simulink model "boundingbox"  (R2018a)
settings: Solver=VariableStepAuto  StartTime=0.0  StopTime=10.0  RelTol=1e-3
libraries: simulink x128
(part 2 of 4)

== system boundingbox/generate_proximity_sensor_readings/Subsystem/distance_to_bounding_box ==
  note: bounding rectangle
      | C---D
      | |  >  |
      | B---A
  "vertex_a " : Inport
  vertex_b : Inport  Port=2
  vertex_c : Inport  Port=3
  vertex_d : Inport  Port=4
  sensor_pos : Inport  Port=5
  "sensor_ray " : Inport  Port=6
  Inf{,1..3} (4 alike) : Constant  Value=inf
  Min : MinMax  Inputs=4
  Switch{,1..3} (4 alike) : Switch  Criteria=u2 > Threshold
  "calculate_intersection " : Subsystem
  calculate_intersection 1 : Subsystem
  calculate_intersection 2 : Subsystem
  calculate_intersection 3 : Subsystem
  distance : Outport
  wires:
  "vertex_a "/1 -> calculate_intersection 3/2(vertex_2), "calculate_intersection "/1(vertex_1)
  vertex_b/1 -> calculate_intersection 1/1(vertex_1), "calculate_intersection "/2(vertex_2)
  vertex_c/1 -> calculate_intersection 2/1(vertex_1), calculate_intersection 1/2(vertex_2)
  vertex_d/1 -> calculate_intersection 3/1(vertex_1), calculate_intersection 2/2(vertex_2)
  sensor_pos/1 -> calculate_intersection 3/3("origin "), calculate_intersection 2/3("origin "), calculate_intersection 1/3("origin "), "calculate_intersection "/3("origin ")
  "sensor_ray "/1 -> calculate_intersection 3/4(ray), calculate_intersection 2/4(ray), calculate_intersection 1/4(ray), "calculate_intersection "/4(ray)
  "calculate_intersection "/2(intersection (0,1)) -> Switch/2
  Inf/1 -> Switch/3
  Inf1/1 -> Switch1/3
  calculate_intersection 1/2(intersection (0,1)) -> Switch1/2
  calculate_intersection 2/2(intersection (0,1)) -> Switch2/2
  calculate_intersection 3/2(intersection (0,1)) -> Switch3/2
  Inf2/1 -> Switch2/3
  Inf3/1 -> Switch3/3
  calculate_intersection 3/1(distance) -> Switch3/1
  calculate_intersection 2/1(distance) -> Switch2/1
  calculate_intersection 1/1(distance) -> Switch1/1
  "calculate_intersection "/1(distance) -> Switch/1
  Switch/1 -> Min/1
  Switch1/1 -> Min/2
  Switch2/1 -> Min/3
  Switch3/1 -> Min/4
  Min/1 -> distance/1

== system boundingbox/generate_proximity_sensor_readings/Subsystem/distance_to_bounding_box1 ==
  note: bounding rectangle
      | C---D
      | |  >  |
      | B---A
  "vertex_a " : Inport
  vertex_b : Inport  Port=2
  vertex_c : Inport  Port=3
  vertex_d : Inport  Port=4
  sensor_pos : Inport  Port=5
  "sensor_ray " : Inport  Port=6
  Inf{,1..3} (4 alike) : Constant  Value=inf
  Min : MinMax  Inputs=4
  Switch{,1..3} (4 alike) : Switch  Criteria=u2 > Threshold
  "calculate_intersection " : Subsystem
  calculate_intersection 1 : Subsystem
  calculate_intersection 2 : Subsystem
  calculate_intersection 3 : Subsystem
  distance : Outport
  wires:
  Min/1 -> distance/1
  Switch3/1 -> Min/4
  Switch2/1 -> Min/3
  Switch1/1 -> Min/2
  Switch/1 -> Min/1
  "calculate_intersection "/1(distance) -> Switch/1
  calculate_intersection 1/1(distance) -> Switch1/1
  calculate_intersection 2/1(distance) -> Switch2/1
  calculate_intersection 3/1(distance) -> Switch3/1
  Inf3/1 -> Switch3/3
  Inf2/1 -> Switch2/3
  calculate_intersection 3/2(intersection (0,1)) -> Switch3/2
  calculate_intersection 2/2(intersection (0,1)) -> Switch2/2
  calculate_intersection 1/2(intersection (0,1)) -> Switch1/2
  Inf1/1 -> Switch1/3
  Inf/1 -> Switch/3
  "calculate_intersection "/2(intersection (0,1)) -> Switch/2
  "sensor_ray "/1 -> calculate_intersection 3/4(ray), calculate_intersection 2/4(ray), calculate_intersection 1/4(ray), "calculate_intersection "/4(ray)
  sensor_pos/1 -> calculate_intersection 3/3("origin "), calculate_intersection 2/3("origin "), calculate_intersection 1/3("origin "), "calculate_intersection "/3("origin ")
  vertex_d/1 -> calculate_intersection 3/1(vertex_1), calculate_intersection 2/2(vertex_2)
  vertex_c/1 -> calculate_intersection 2/1(vertex_1), calculate_intersection 1/2(vertex_2)
  vertex_b/1 -> calculate_intersection 1/1(vertex_1), "calculate_intersection "/2(vertex_2)
  "vertex_a "/1 -> calculate_intersection 3/2(vertex_2), "calculate_intersection "/1(vertex_1)

== system boundingbox/generate_proximity_sensor_readings/Subsystem/distance_to_bounding_box2 ==
  note: bounding rectangle
      | C---D
      | |  >  |
      | B---A
  "vertex_a " : Inport
  vertex_b : Inport  Port=2
  vertex_c : Inport  Port=3
  vertex_d : Inport  Port=4
  sensor_pos : Inport  Port=5
  "sensor_ray " : Inport  Port=6
  Inf{,1..3} (4 alike) : Constant  Value=inf
  Min : MinMax  Inputs=4
  Switch{,1..3} (4 alike) : Switch  Criteria=u2 > Threshold
  "calculate_intersection " : Subsystem
  calculate_intersection 1 : Subsystem
  calculate_intersection 2 : Subsystem
  calculate_intersection 3 : Subsystem
  distance : Outport
  wires:
  "vertex_a "/1 -> calculate_intersection 3/2(vertex_2), "calculate_intersection "/1(vertex_1)
  vertex_b/1 -> calculate_intersection 1/1(vertex_1), "calculate_intersection "/2(vertex_2)
  vertex_c/1 -> calculate_intersection 2/1(vertex_1), calculate_intersection 1/2(vertex_2)
  vertex_d/1 -> calculate_intersection 3/1(vertex_1), calculate_intersection 2/2(vertex_2)
  sensor_pos/1 -> calculate_intersection 3/3("origin "), calculate_intersection 2/3("origin "), calculate_intersection 1/3("origin "), "calculate_intersection "/3("origin ")
  "sensor_ray "/1 -> calculate_intersection 3/4(ray), calculate_intersection 2/4(ray), calculate_intersection 1/4(ray), "calculate_intersection "/4(ray)
  "calculate_intersection "/2(intersection (0,1)) -> Switch/2
  Inf/1 -> Switch/3
  Inf1/1 -> Switch1/3
  calculate_intersection 1/2(intersection (0,1)) -> Switch1/2
  calculate_intersection 2/2(intersection (0,1)) -> Switch2/2
  calculate_intersection 3/2(intersection (0,1)) -> Switch3/2
  Inf2/1 -> Switch2/3
  Inf3/1 -> Switch3/3
  calculate_intersection 3/1(distance) -> Switch3/1
  calculate_intersection 2/1(distance) -> Switch2/1
  calculate_intersection 1/1(distance) -> Switch1/1
  "calculate_intersection "/1(distance) -> Switch/1
  Switch/1 -> Min/1
  Switch1/1 -> Min/2
  Switch2/1 -> Min/3
  Switch3/1 -> Min/4
  Min/1 -> distance/1

== system boundingbox/generate_proximity_sensor_readings/Subsystem/distance_to_proximity_sensor_data  ==
  distance_cm : Inport
  Constant : Constant  Value=0
  Constant1 : Constant  Value=255
  Gain : Gain  Gain=255/30
  Max : MinMax  Function=max  Inputs=2
  Subtract : Sum  Inputs=+-
  "prox_sensor_input " : Outport
  wires:
  distance_cm/1 -> Gain/1
  Gain/1 -> Subtract/2
  Subtract/1 -> Max/2
  Constant/1 -> Max/1
  Max/1 -> "prox_sensor_input "/1
  Constant1/1 -> Subtract/1

== system boundingbox/generate_proximity_sensor_readings/Subsystem1/distance_to_bounding_box ==
  note: bounding rectangle
      | C---D
      | |  >  |
      | B---A
  "vertex_a " : Inport
  vertex_b : Inport  Port=2
  vertex_c : Inport  Port=3
  vertex_d : Inport  Port=4
  sensor_pos : Inport  Port=5
  "sensor_ray " : Inport  Port=6
  Inf{,1..3} (4 alike) : Constant  Value=inf
  Min : MinMax  Inputs=4
  Switch{,1..3} (4 alike) : Switch  Criteria=u2 > Threshold
  "calculate_intersection " : Subsystem
  calculate_intersection 1 : Subsystem
  calculate_intersection 2 : Subsystem
  calculate_intersection 3 : Subsystem
  distance : Outport
  wires:
  Min/1 -> distance/1
  Switch3/1 -> Min/4
  Switch2/1 -> Min/3
  Switch1/1 -> Min/2
  Switch/1 -> Min/1
  "calculate_intersection "/1(distance) -> Switch/1
  calculate_intersection 1/1(distance) -> Switch1/1
  calculate_intersection 2/1(distance) -> Switch2/1
  calculate_intersection 3/1(distance) -> Switch3/1
  Inf3/1 -> Switch3/3
  Inf2/1 -> Switch2/3
  calculate_intersection 3/2(intersection (0,1)) -> Switch3/2
  calculate_intersection 2/2(intersection (0,1)) -> Switch2/2
  calculate_intersection 1/2(intersection (0,1)) -> Switch1/2
  Inf1/1 -> Switch1/3
  Inf/1 -> Switch/3
  "calculate_intersection "/2(intersection (0,1)) -> Switch/2
  "sensor_ray "/1 -> calculate_intersection 3/4(ray), calculate_intersection 2/4(ray), calculate_intersection 1/4(ray), "calculate_intersection "/4(ray)
  sensor_pos/1 -> calculate_intersection 3/3("origin "), calculate_intersection 2/3("origin "), calculate_intersection 1/3("origin "), "calculate_intersection "/3("origin ")
  vertex_d/1 -> calculate_intersection 3/1(vertex_1), calculate_intersection 2/2(vertex_2)
  vertex_c/1 -> calculate_intersection 2/1(vertex_1), calculate_intersection 1/2(vertex_2)
  vertex_b/1 -> calculate_intersection 1/1(vertex_1), "calculate_intersection "/2(vertex_2)
  "vertex_a "/1 -> calculate_intersection 3/2(vertex_2), "calculate_intersection "/1(vertex_1)

== system boundingbox/generate_proximity_sensor_readings/Subsystem1/distance_to_bounding_box1 ==
  note: bounding rectangle
      | C---D
      | |  >  |
      | B---A
  "vertex_a " : Inport
  vertex_b : Inport  Port=2
  vertex_c : Inport  Port=3
  vertex_d : Inport  Port=4
  sensor_pos : Inport  Port=5
  "sensor_ray " : Inport  Port=6
  Inf{,1..3} (4 alike) : Constant  Value=inf
  Min : MinMax  Inputs=4
  Switch{,1..3} (4 alike) : Switch  Criteria=u2 > Threshold
  "calculate_intersection " : Subsystem
  calculate_intersection 1 : Subsystem
  calculate_intersection 2 : Subsystem
  calculate_intersection 3 : Subsystem
  distance : Outport
  wires:
  "vertex_a "/1 -> calculate_intersection 3/2(vertex_2), "calculate_intersection "/1(vertex_1)
  vertex_b/1 -> calculate_intersection 1/1(vertex_1), "calculate_intersection "/2(vertex_2)
  vertex_c/1 -> calculate_intersection 2/1(vertex_1), calculate_intersection 1/2(vertex_2)
  vertex_d/1 -> calculate_intersection 3/1(vertex_1), calculate_intersection 2/2(vertex_2)
  sensor_pos/1 -> calculate_intersection 3/3("origin "), calculate_intersection 2/3("origin "), calculate_intersection 1/3("origin "), "calculate_intersection "/3("origin ")
  "sensor_ray "/1 -> calculate_intersection 3/4(ray), calculate_intersection 2/4(ray), calculate_intersection 1/4(ray), "calculate_intersection "/4(ray)
  "calculate_intersection "/2(intersection (0,1)) -> Switch/2
  Inf/1 -> Switch/3
  Inf1/1 -> Switch1/3
  calculate_intersection 1/2(intersection (0,1)) -> Switch1/2
  calculate_intersection 2/2(intersection (0,1)) -> Switch2/2
  calculate_intersection 3/2(intersection (0,1)) -> Switch3/2
  Inf2/1 -> Switch2/3
  Inf3/1 -> Switch3/3
  calculate_intersection 3/1(distance) -> Switch3/1
  calculate_intersection 2/1(distance) -> Switch2/1
  calculate_intersection 1/1(distance) -> Switch1/1
  "calculate_intersection "/1(distance) -> Switch/1
  Switch/1 -> Min/1
  Switch1/1 -> Min/2
  Switch2/1 -> Min/3
  Switch3/1 -> Min/4
  Min/1 -> distance/1

== system boundingbox/generate_proximity_sensor_readings/Subsystem1/distance_to_bounding_box2 ==
  note: bounding rectangle
      | C---D
      | |  >  |
      | B---A
  "vertex_a " : Inport
  vertex_b : Inport  Port=2
  vertex_c : Inport  Port=3
  vertex_d : Inport  Port=4
  sensor_pos : Inport  Port=5
  "sensor_ray " : Inport  Port=6
  Inf{,1..3} (4 alike) : Constant  Value=inf
  Min : MinMax  Inputs=4
  Switch{,1..3} (4 alike) : Switch  Criteria=u2 > Threshold
  "calculate_intersection " : Subsystem
  calculate_intersection 1 : Subsystem
  calculate_intersection 2 : Subsystem
  calculate_intersection 3 : Subsystem
  distance : Outport
  wires:
  Min/1 -> distance/1
  Switch3/1 -> Min/4
  Switch2/1 -> Min/3
  Switch1/1 -> Min/2
  Switch/1 -> Min/1
  "calculate_intersection "/1(distance) -> Switch/1
  calculate_intersection 1/1(distance) -> Switch1/1
  calculate_intersection 2/1(distance) -> Switch2/1
  calculate_intersection 3/1(distance) -> Switch3/1
  Inf3/1 -> Switch3/3
  Inf2/1 -> Switch2/3
  calculate_intersection 3/2(intersection (0,1)) -> Switch3/2
  calculate_intersection 2/2(intersection (0,1)) -> Switch2/2
  calculate_intersection 1/2(intersection (0,1)) -> Switch1/2
  Inf1/1 -> Switch1/3
  Inf/1 -> Switch/3
  "calculate_intersection "/2(intersection (0,1)) -> Switch/2
  "sensor_ray "/1 -> calculate_intersection 3/4(ray), calculate_intersection 2/4(ray), calculate_intersection 1/4(ray), "calculate_intersection "/4(ray)
  sensor_pos/1 -> calculate_intersection 3/3("origin "), calculate_intersection 2/3("origin "), calculate_intersection 1/3("origin "), "calculate_intersection "/3("origin ")
  vertex_d/1 -> calculate_intersection 3/1(vertex_1), calculate_intersection 2/2(vertex_2)
  vertex_c/1 -> calculate_intersection 2/1(vertex_1), calculate_intersection 1/2(vertex_2)
  vertex_b/1 -> calculate_intersection 1/1(vertex_1), "calculate_intersection "/2(vertex_2)
  "vertex_a "/1 -> calculate_intersection 3/2(vertex_2), "calculate_intersection "/1(vertex_1)

== system boundingbox/generate_proximity_sensor_readings/Subsystem1/distance_to_proximity_sensor_data  ==
  distance_cm : Inport
  Constant : Constant  Value=0
  Constant1 : Constant  Value=255
  Gain : Gain  Gain=255/30
  Max : MinMax  Function=max  Inputs=2
  Subtract : Sum  Inputs=+-
  "prox_sensor_input " : Outport
  wires:
  Constant1/1 -> Subtract/1
  Max/1 -> "prox_sensor_input "/1
  Constant/1 -> Max/1
  Subtract/1 -> Max/2
  Gain/1 -> Subtract/2
  distance_cm/1 -> Gain/1

== system boundingbox/generate_proximity_sensor_readings/Subsystem2/distance_to_bounding_box ==
  note: bounding rectangle
      | C---D
      | |  >  |
      | B---A
  "vertex_a " : Inport
  vertex_b : Inport  Port=2
  vertex_c : Inport  Port=3
  vertex_d : Inport  Port=4
  sensor_pos : Inport  Port=5
  "sensor_ray " : Inport  Port=6
  Inf{,1..3} (4 alike) : Constant  Value=inf
  Min : MinMax  Inputs=4
  Switch{,1..3} (4 alike) : Switch  Criteria=u2 > Threshold
  "calculate_intersection " : Subsystem
  calculate_intersection 1 : Subsystem
  calculate_intersection 2 : Subsystem
  calculate_intersection 3 : Subsystem
  distance : Outport
  wires:
  "vertex_a "/1 -> calculate_intersection 3/2(vertex_2), "calculate_intersection "/1(vertex_1)
  vertex_b/1 -> calculate_intersection 1/1(vertex_1), "calculate_intersection "/2(vertex_2)
  vertex_c/1 -> calculate_intersection 2/1(vertex_1), calculate_intersection 1/2(vertex_2)
  vertex_d/1 -> calculate_intersection 3/1(vertex_1), calculate_intersection 2/2(vertex_2)
  sensor_pos/1 -> calculate_intersection 3/3("origin "), calculate_intersection 2/3("origin "), calculate_intersection 1/3("origin "), "calculate_intersection "/3("origin ")
  "sensor_ray "/1 -> calculate_intersection 3/4(ray), calculate_intersection 2/4(ray), calculate_intersection 1/4(ray), "calculate_intersection "/4(ray)
  "calculate_intersection "/2(intersection (0,1)) -> Switch/2
  Inf/1 -> Switch/3
  Inf1/1 -> Switch1/3
  calculate_intersection 1/2(intersection (0,1)) -> Switch1/2
  calculate_intersection 2/2(intersection (0,1)) -> Switch2/2
  calculate_intersection 3/2(intersection (0,1)) -> Switch3/2
  Inf2/1 -> Switch2/3
  Inf3/1 -> Switch3/3
  calculate_intersection 3/1(distance) -> Switch3/1
  calculate_intersection 2/1(distance) -> Switch2/1
  calculate_intersection 1/1(distance) -> Switch1/1
  "calculate_intersection "/1(distance) -> Switch/1
  Switch/1 -> Min/1
  Switch1/1 -> Min/2
  Switch2/1 -> Min/3
  Switch3/1 -> Min/4
  Min/1 -> distance/1

== system boundingbox/generate_proximity_sensor_readings/Subsystem2/distance_to_bounding_box1 ==
  note: bounding rectangle
      | C---D
      | |  >  |
      | B---A
  "vertex_a " : Inport
  vertex_b : Inport  Port=2
  vertex_c : Inport  Port=3
  vertex_d : Inport  Port=4
  sensor_pos : Inport  Port=5
  "sensor_ray " : Inport  Port=6
  Inf{,1..3} (4 alike) : Constant  Value=inf
  Min : MinMax  Inputs=4
  Switch{,1..3} (4 alike) : Switch  Criteria=u2 > Threshold
  "calculate_intersection " : Subsystem
  calculate_intersection 1 : Subsystem
  calculate_intersection 2 : Subsystem
  calculate_intersection 3 : Subsystem
  distance : Outport
  wires:
  Min/1 -> distance/1
  Switch3/1 -> Min/4
  Switch2/1 -> Min/3
  Switch1/1 -> Min/2
  Switch/1 -> Min/1
  "calculate_intersection "/1(distance) -> Switch/1
  calculate_intersection 1/1(distance) -> Switch1/1
  calculate_intersection 2/1(distance) -> Switch2/1
  calculate_intersection 3/1(distance) -> Switch3/1
  Inf3/1 -> Switch3/3
  Inf2/1 -> Switch2/3
  calculate_intersection 3/2(intersection (0,1)) -> Switch3/2
  calculate_intersection 2/2(intersection (0,1)) -> Switch2/2
  calculate_intersection 1/2(intersection (0,1)) -> Switch1/2
  Inf1/1 -> Switch1/3
  Inf/1 -> Switch/3
  "calculate_intersection "/2(intersection (0,1)) -> Switch/2
  "sensor_ray "/1 -> calculate_intersection 3/4(ray), calculate_intersection 2/4(ray), calculate_intersection 1/4(ray), "calculate_intersection "/4(ray)
  sensor_pos/1 -> calculate_intersection 3/3("origin "), calculate_intersection 2/3("origin "), calculate_intersection 1/3("origin "), "calculate_intersection "/3("origin ")
  vertex_d/1 -> calculate_intersection 3/1(vertex_1), calculate_intersection 2/2(vertex_2)
  vertex_c/1 -> calculate_intersection 2/1(vertex_1), calculate_intersection 1/2(vertex_2)
  vertex_b/1 -> calculate_intersection 1/1(vertex_1), "calculate_intersection "/2(vertex_2)
  "vertex_a "/1 -> calculate_intersection 3/2(vertex_2), "calculate_intersection "/1(vertex_1)

== system boundingbox/generate_proximity_sensor_readings/Subsystem2/distance_to_bounding_box2 ==
  note: bounding rectangle
      | C---D
      | |  >  |
      | B---A
  "vertex_a " : Inport
  vertex_b : Inport  Port=2
  vertex_c : Inport  Port=3
  vertex_d : Inport  Port=4
  sensor_pos : Inport  Port=5
  "sensor_ray " : Inport  Port=6
  Inf{,1..3} (4 alike) : Constant  Value=inf
  Min : MinMax  Inputs=4
  Switch{,1..3} (4 alike) : Switch  Criteria=u2 > Threshold
  "calculate_intersection " : Subsystem
  calculate_intersection 1 : Subsystem
  calculate_intersection 2 : Subsystem
  calculate_intersection 3 : Subsystem
  distance : Outport
  wires:
  "vertex_a "/1 -> calculate_intersection 3/2(vertex_2), "calculate_intersection "/1(vertex_1)
  vertex_b/1 -> calculate_intersection 1/1(vertex_1), "calculate_intersection "/2(vertex_2)
  vertex_c/1 -> calculate_intersection 2/1(vertex_1), calculate_intersection 1/2(vertex_2)
  vertex_d/1 -> calculate_intersection 3/1(vertex_1), calculate_intersection 2/2(vertex_2)
  sensor_pos/1 -> calculate_intersection 3/3("origin "), calculate_intersection 2/3("origin "), calculate_intersection 1/3("origin "), "calculate_intersection "/3("origin ")
  "sensor_ray "/1 -> calculate_intersection 3/4(ray), calculate_intersection 2/4(ray), calculate_intersection 1/4(ray), "calculate_intersection "/4(ray)
  "calculate_intersection "/2(intersection (0,1)) -> Switch/2
  Inf/1 -> Switch/3
  Inf1/1 -> Switch1/3
  calculate_intersection 1/2(intersection (0,1)) -> Switch1/2
  calculate_intersection 2/2(intersection (0,1)) -> Switch2/2
  calculate_intersection 3/2(intersection (0,1)) -> Switch3/2
  Inf2/1 -> Switch2/3
  Inf3/1 -> Switch3/3
  calculate_intersection 3/1(distance) -> Switch3/1
  calculate_intersection 2/1(distance) -> Switch2/1
  calculate_intersection 1/1(distance) -> Switch1/1
  "calculate_intersection "/1(distance) -> Switch/1
  Switch/1 -> Min/1
  Switch1/1 -> Min/2
  Switch2/1 -> Min/3
  Switch3/1 -> Min/4
  Min/1 -> distance/1

== system boundingbox/generate_proximity_sensor_readings/Subsystem2/distance_to_proximity_sensor_data  ==
  distance_cm : Inport
  Constant : Constant  Value=0
  Constant1 : Constant  Value=255
  Gain : Gain  Gain=255/30
  Max : MinMax  Function=max  Inputs=2
  Subtract : Sum  Inputs=+-
  "prox_sensor_input " : Outport
  wires:
  distance_cm/1 -> Gain/1
  Gain/1 -> Subtract/2
  Subtract/1 -> Max/2
  Constant/1 -> Max/1
  Max/1 -> "prox_sensor_input "/1
  Constant1/1 -> Subtract/1

== system boundingbox/generate_proximity_sensor_readings/bounding_box_CollectorB/vector rotation  ==
  angle : Inport
  x_dir : Inport  Port=2
  y_dir : Inport  Port=3
  Cos : Trigonometry  Operator=cos
  Multiply{,1..3} (4 alike) : Product
  Sin : Trigonometry
  Subtract : Sum  Inputs=+-
  Subtract1 : Sum
  Vector Concatenate1 : Concatenate
  "rotated_vector " : Outport
  wires:
  Multiply2/1 -> Subtract/2
  Subtract/1 -> Vector Concatenate1/1
  Vector Concatenate1/1 -> "rotated_vector "/1
  x_dir/1 -> Multiply/1, Multiply1/1
  angle/1 -> Sin/1, Cos/1
  Sin/1 -> Multiply2/2, Multiply1/2
  Cos/1 -> Multiply/2, Multiply3/2
  Subtract1/1 -> Vector Concatenate1/2
  y_dir/1 -> Multiply2/1, Multiply3/1
  Multiply/1 -> Subtract/1
  Multiply1/1 -> Subtract1/1
  Multiply3/1 -> Subtract1/2

== system boundingbox/generate_proximity_sensor_readings/bounding_box_CollectorB/vector rotation 1 ==
  angle : Inport
  x_dir : Inport  Port=2
  y_dir : Inport  Port=3
  Cos : Trigonometry  Operator=cos
  Multiply{,1..3} (4 alike) : Product
  Sin : Trigonometry
  Subtract : Sum  Inputs=+-
  Subtract1 : Sum
  Vector Concatenate1 : Concatenate
  "rotated_vector " : Outport
  wires:
  Multiply3/1 -> Subtract1/2
  Multiply1/1 -> Subtract1/1
  Multiply/1 -> Subtract/1
  y_dir/1 -> Multiply3/1, Multiply2/1
  Subtract1/1 -> Vector Concatenate1/2
  Cos/1 -> Multiply3/2, Multiply/2
  Sin/1 -> Multiply1/2, Multiply2/2
  angle/1 -> Cos/1, Sin/1
  x_dir/1 -> Multiply1/1, Multiply/1
  Vector Concatenate1/1 -> "rotated_vector "/1
  Subtract/1 -> Vector Concatenate1/1
  Multiply2/1 -> Subtract/2

== system boundingbox/generate_proximity_sensor_readings/bounding_box_ScoutA/vector rotation  ==
  angle : Inport
  x_dir : Inport  Port=2
  y_dir : Inport  Port=3
  Cos : Trigonometry  Operator=cos
  Multiply{,1..3} (4 alike) : Product
  Sin : Trigonometry
  Subtract : Sum  Inputs=+-
  Subtract1 : Sum
  Vector Concatenate1 : Concatenate
  "rotated_vector " : Outport
  wires:
  Multiply2/1 -> Subtract/2
  Subtract/1 -> Vector Concatenate1/1
  Vector Concatenate1/1 -> "rotated_vector "/1
  x_dir/1 -> Multiply/1, Multiply1/1
  angle/1 -> Sin/1, Cos/1
  Sin/1 -> Multiply2/2, Multiply1/2
  Cos/1 -> Multiply/2, Multiply3/2
  Subtract1/1 -> Vector Concatenate1/2
  y_dir/1 -> Multiply2/1, Multiply3/1
  Multiply/1 -> Subtract/1
  Multiply1/1 -> Subtract1/1
  Multiply3/1 -> Subtract1/2

== system boundingbox/generate_proximity_sensor_readings/bounding_box_ScoutA/vector rotation 1 ==
  angle : Inport
  x_dir : Inport  Port=2
  y_dir : Inport  Port=3
  Cos : Trigonometry  Operator=cos
  Multiply{,1..3} (4 alike) : Product
  Sin : Trigonometry
  Subtract : Sum  Inputs=+-
  Subtract1 : Sum
  Vector Concatenate1 : Concatenate
  "rotated_vector " : Outport
  wires:
  Multiply3/1 -> Subtract1/2
  Multiply1/1 -> Subtract1/1
  Multiply/1 -> Subtract/1
  y_dir/1 -> Multiply3/1, Multiply2/1
  Subtract1/1 -> Vector Concatenate1/2
  Cos/1 -> Multiply3/2, Multiply/2
  Sin/1 -> Multiply1/2, Multiply2/2
  angle/1 -> Cos/1, Sin/1
  x_dir/1 -> Multiply1/1, Multiply/1
  Vector Concatenate1/1 -> "rotated_vector "/1
  Subtract/1 -> Vector Concatenate1/1
  Multiply2/1 -> Subtract/2

== system boundingbox/generate_proximity_sensor_readings/bounding_box_ScoutB/vector rotation  ==
  angle : Inport
  x_dir : Inport  Port=2
  y_dir : Inport  Port=3
  Cos : Trigonometry  Operator=cos
  Multiply{,1..3} (4 alike) : Product
  Sin : Trigonometry
  Subtract : Sum  Inputs=+-
  Subtract1 : Sum
  Vector Concatenate1 : Concatenate
  "rotated_vector " : Outport
  wires:
  Multiply3/1 -> Subtract1/2
  Multiply1/1 -> Subtract1/1
  Multiply/1 -> Subtract/1
  y_dir/1 -> Multiply3/1, Multiply2/1
  Subtract1/1 -> Vector Concatenate1/2
  Cos/1 -> Multiply3/2, Multiply/2
  Sin/1 -> Multiply1/2, Multiply2/2
  angle/1 -> Cos/1, Sin/1
  x_dir/1 -> Multiply1/1, Multiply/1
  Vector Concatenate1/1 -> "rotated_vector "/1
  Subtract/1 -> Vector Concatenate1/1
  Multiply2/1 -> Subtract/2

== system boundingbox/generate_proximity_sensor_readings/bounding_box_ScoutB/vector rotation 1 ==
  angle : Inport
  x_dir : Inport  Port=2
  y_dir : Inport  Port=3
  Cos : Trigonometry  Operator=cos
  Multiply{,1..3} (4 alike) : Product
  Sin : Trigonometry
  Subtract : Sum  Inputs=+-
  Subtract1 : Sum
  Vector Concatenate1 : Concatenate
  "rotated_vector " : Outport
  wires:
  Multiply2/1 -> Subtract/2
  Subtract/1 -> Vector Concatenate1/1
  Vector Concatenate1/1 -> "rotated_vector "/1
  x_dir/1 -> Multiply/1, Multiply1/1
  angle/1 -> Sin/1, Cos/1
  Sin/1 -> Multiply2/2, Multiply1/2
  Cos/1 -> Multiply/2, Multiply3/2
  Subtract1/1 -> Vector Concatenate1/2
  y_dir/1 -> Multiply2/1, Multiply3/1
  Multiply/1 -> Subtract/1
  Multiply1/1 -> Subtract1/1
  Multiply3/1 -> Subtract1/2

== system boundingbox/generate_proximity_sensor_readings/sensor_ray_generation front/vector rotation  ==
  angle : Inport
  x_dir : Inport  Port=2
  y_dir : Inport  Port=3
  Cos : Trigonometry  Operator=cos
  Multiply{,1..3} (4 alike) : Product
  Sin : Trigonometry
  Subtract : Sum  Inputs=+-
  Subtract1 : Sum
  Vector Concatenate1 : Concatenate
  "rotated_vector " : Outport
  wires:
  Multiply3/1 -> Subtract1/2
  Multiply1/1 -> Subtract1/1
  Multiply/1 -> Subtract/1
  y_dir/1 -> Multiply3/1, Multiply2/1
  Subtract1/1 -> Vector Concatenate1/2
  Cos/1 -> Multiply3/2, Multiply/2
  Sin/1 -> Multiply1/2, Multiply2/2
  angle/1 -> Cos/1, Sin/1
  x_dir/1 -> Multiply1/1, Multiply/1
  Vector Concatenate1/1 -> "rotated_vector "/1
  Subtract/1 -> Vector Concatenate1/1
  Multiply2/1 -> Subtract/2

== system boundingbox/generate_proximity_sensor_readings/sensor_ray_generation left/vector rotation  ==
  angle : Inport
  x_dir : Inport  Port=2
  y_dir : Inport  Port=3
  Cos : Trigonometry  Operator=cos
  Multiply{,1..3} (4 alike) : Product
  Sin : Trigonometry
  Subtract : Sum  Inputs=+-
  Subtract1 : Sum
  Vector Concatenate1 : Concatenate
  "rotated_vector " : Outport
  wires:
  Multiply2/1 -> Subtract/2
  Subtract/1 -> Vector Concatenate1/1
  Vector Concatenate1/1 -> "rotated_vector "/1
  x_dir/1 -> Multiply/1, Multiply1/1
  angle/1 -> Sin/1, Cos/1
  Sin/1 -> Multiply2/2, Multiply1/2
  Cos/1 -> Multiply/2, Multiply3/2
  Subtract1/1 -> Vector Concatenate1/2
  y_dir/1 -> Multiply2/1, Multiply3/1
  Multiply/1 -> Subtract/1
  Multiply1/1 -> Subtract1/1
  Multiply3/1 -> Subtract1/2

== system boundingbox/generate_proximity_sensor_readings/sensor_ray_generation right/vector rotation  ==
  angle : Inport
  x_dir : Inport  Port=2
  y_dir : Inport  Port=3
  Cos : Trigonometry  Operator=cos
  Multiply{,1..3} (4 alike) : Product
  Sin : Trigonometry
  Subtract : Sum  Inputs=+-
  Subtract1 : Sum
  Vector Concatenate1 : Concatenate
  "rotated_vector " : Outport
  wires:
  Multiply3/1 -> Subtract1/2
  Multiply1/1 -> Subtract1/1
  Multiply/1 -> Subtract/1
  y_dir/1 -> Multiply3/1, Multiply2/1
  Subtract1/1 -> Vector Concatenate1/2
  Cos/1 -> Multiply3/2, Multiply/2
  Sin/1 -> Multiply1/2, Multiply2/2
  angle/1 -> Cos/1, Sin/1
  x_dir/1 -> Multiply1/1, Multiply/1
  Vector Concatenate1/1 -> "rotated_vector "/1
  Subtract/1 -> Vector Concatenate1/1
  Multiply2/1 -> Subtract/2

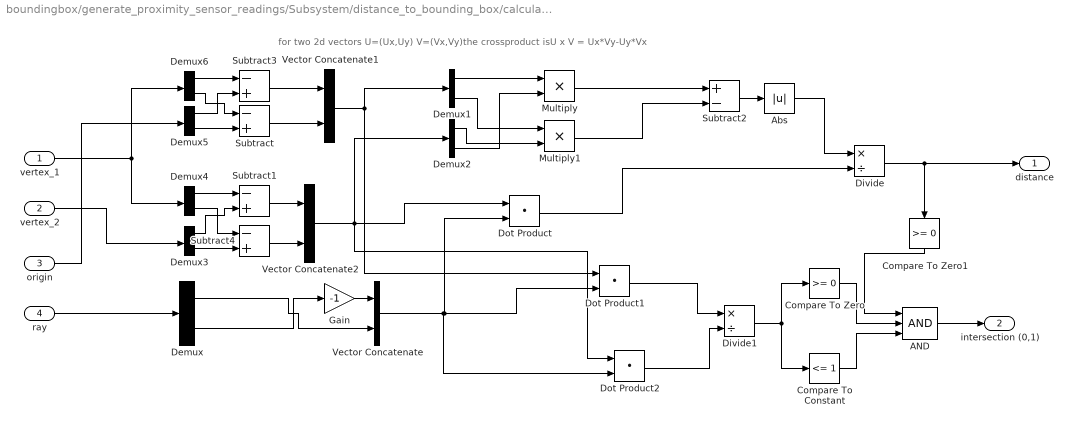
== system boundingbox/generate_proximity_sensor_readings/Subsystem/distance_to_bounding_box/calculate_intersection  ==
  note: for two 2d vectors U=(Ux,Uy) V=(Vx,Vy)the crossproduct isU x V = Ux*Vy-Uy*Vx
  vertex_1 : Inport
  vertex_2 : Inport  Port=2
  "origin " : Inport  Port=3
  ray : Inport  Port=4
  AND : Logic  Inputs=3  IconShape=distinctive  AllPortsSameDT=off  OutDataTypeStr=boolean
  Abs : Abs
  Compare To Constant : simulink/Logic and Bit Operations/Compare To Constant  relop=<=  const=1  OutDataTypeStr=boolean
  Compare To Zero : simulink/Logic and Bit Operations/Compare To Zero  relop=>=  OutDataTypeStr=boolean
  Compare To Zero1 : simulink/Logic and Bit Operations/Compare To Zero  relop=>=  OutDataTypeStr=boolean
  Demux{,1..6} (7 alike) : Demux  Outputs=2
  Divide : Product  Inputs=*/
  Divide1 : Product  Inputs=*/
  Dot Product : DotProduct  InputSameDT=on  OutDataTypeStr=Inherit: Inherit via internal rule
  Dot Product1 : DotProduct  InputSameDT=on  OutDataTypeStr=Inherit: Inherit via internal rule
  Dot Product2 : DotProduct  InputSameDT=on  OutDataTypeStr=Inherit: Inherit via internal rule
  Gain : Gain  Gain=-1
  Multiply : Product
  Multiply1 : Product
  Subtract{,1,3..4} (4 alike) : Sum  Inputs=-+
  Subtract2 : Sum  Inputs=+-
  Vector Concatenate : Concatenate
  Vector Concatenate1 : Concatenate
  Vector Concatenate2 : Concatenate
  distance : Outport
  intersection (0,1) : Outport  Port=2
  wires:
  Compare To Constant/1 -> AND/3
  Compare To Zero/1 -> AND/2
  Divide1/1 -> Compare To Zero/1, Compare To Constant/1
  AND/1 -> intersection (0,1)/1
  Dot Product2/1 -> Divide1/2
  Dot Product1/1 -> Divide1/1
  Multiply1/1 -> Subtract2/2
  Multiply/1 -> Subtract2/1
  Demux2/1 -> Multiply1/2
  Demux1/2 -> Multiply1/1
  Demux2/2 -> Multiply/2
  Demux1/1 -> Multiply/1
  Abs/1 -> Divide/1
  Subtract2/1 -> Abs/1
  Dot Product/1 -> Divide/2
  Divide/1 -> Compare To Zero1/1, distance/1
  Subtract/1 -> Vector Concatenate1/2
  Vector Concatenate/1 -> Dot Product/2, Dot Product1/2, Dot Product2/2
  Demux/1 -> Vector Concatenate/2
  Gain/1 -> Vector Concatenate/1
  Demux/2 -> Gain/1
  ray/1 -> Demux/1
  vertex_2/1 -> Demux3/1
  vertex_1/1 -> Demux6/1, Demux4/1
  "origin "/1 -> Demux5/1
  Demux5/1 -> Subtract3/2
  Demux6/1 -> Subtract3/1
  Demux6/2 -> Subtract/1
  Demux5/2 -> Subtract/2
  Demux4/1 -> Subtract1/1
  Demux4/2 -> Subtract4/1
  Demux3/1 -> Subtract1/2
  Demux3/2 -> Subtract4/2
  Subtract3/1 -> Vector Concatenate1/1
  Vector Concatenate1/1 -> Dot Product1/1, Demux1/1
  Subtract4/1 -> Vector Concatenate2/2
  Subtract1/1 -> Vector Concatenate2/1
  Vector Concatenate2/1 -> Dot Product/1, Demux2/1, Dot Product2/1
  Compare To Zero1/1 -> AND/1

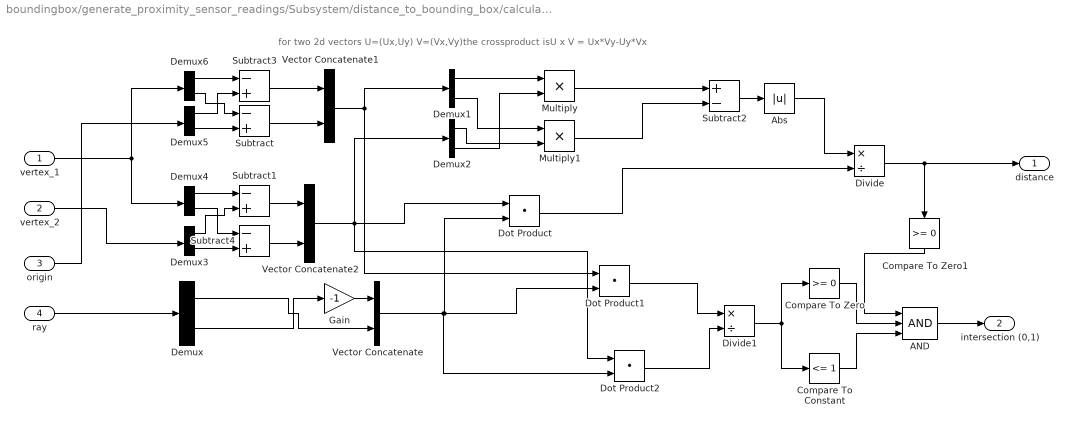
== system boundingbox/generate_proximity_sensor_readings/Subsystem/distance_to_bounding_box/calculate_intersection 1 ==
  note: for two 2d vectors U=(Ux,Uy) V=(Vx,Vy)the crossproduct isU x V = Ux*Vy-Uy*Vx
  vertex_1 : Inport
  vertex_2 : Inport  Port=2
  "origin " : Inport  Port=3
  ray : Inport  Port=4
  AND : Logic  Inputs=3  IconShape=distinctive  AllPortsSameDT=off  OutDataTypeStr=boolean
  Abs : Abs
  Compare To Constant : simulink/Logic and Bit Operations/Compare To Constant  relop=<=  const=1  OutDataTypeStr=boolean
  Compare To Zero : simulink/Logic and Bit Operations/Compare To Zero  relop=>=  OutDataTypeStr=boolean
  Compare To Zero1 : simulink/Logic and Bit Operations/Compare To Zero  relop=>=  OutDataTypeStr=boolean
  Demux{,1..6} (7 alike) : Demux  Outputs=2
  Divide : Product  Inputs=*/
  Divide1 : Product  Inputs=*/
  Dot Product : DotProduct  InputSameDT=on  OutDataTypeStr=Inherit: Inherit via internal rule
  Dot Product1 : DotProduct  InputSameDT=on  OutDataTypeStr=Inherit: Inherit via internal rule
  Dot Product2 : DotProduct  InputSameDT=on  OutDataTypeStr=Inherit: Inherit via internal rule
  Gain : Gain  Gain=-1
  Multiply : Product
  Multiply1 : Product
  Subtract{,1,3..4} (4 alike) : Sum  Inputs=-+
  Subtract2 : Sum  Inputs=+-
  Vector Concatenate : Concatenate
  Vector Concatenate1 : Concatenate
  Vector Concatenate2 : Concatenate
  distance : Outport
  intersection (0,1) : Outport  Port=2
  wires:
  Compare To Zero1/1 -> AND/1
  Vector Concatenate2/1 -> Dot Product2/1, Demux2/1, Dot Product/1
  Subtract1/1 -> Vector Concatenate2/1
  Subtract4/1 -> Vector Concatenate2/2
  Vector Concatenate1/1 -> Demux1/1, Dot Product1/1
  Subtract3/1 -> Vector Concatenate1/1
  Demux3/2 -> Subtract4/2
  Demux3/1 -> Subtract1/2
  Demux4/2 -> Subtract4/1
  Demux4/1 -> Subtract1/1
  Demux5/2 -> Subtract/2
  Demux6/2 -> Subtract/1
  Demux6/1 -> Subtract3/1
  Demux5/1 -> Subtract3/2
  "origin "/1 -> Demux5/1
  vertex_1/1 -> Demux4/1, Demux6/1
  vertex_2/1 -> Demux3/1
  ray/1 -> Demux/1
  Demux/2 -> Gain/1
  Gain/1 -> Vector Concatenate/1
  Demux/1 -> Vector Concatenate/2
  Vector Concatenate/1 -> Dot Product2/2, Dot Product1/2, Dot Product/2
  Subtract/1 -> Vector Concatenate1/2
  Divide/1 -> distance/1, Compare To Zero1/1
  Dot Product/1 -> Divide/2
  Subtract2/1 -> Abs/1
  Abs/1 -> Divide/1
  Demux1/1 -> Multiply/1
  Demux2/2 -> Multiply/2
  Demux1/2 -> Multiply1/1
  Demux2/1 -> Multiply1/2
  Multiply/1 -> Subtract2/1
  Multiply1/1 -> Subtract2/2
  Dot Product1/1 -> Divide1/1
  Dot Product2/1 -> Divide1/2
  AND/1 -> intersection (0,1)/1
  Divide1/1 -> Compare To Constant/1, Compare To Zero/1
  Compare To Zero/1 -> AND/2
  Compare To Constant/1 -> AND/3

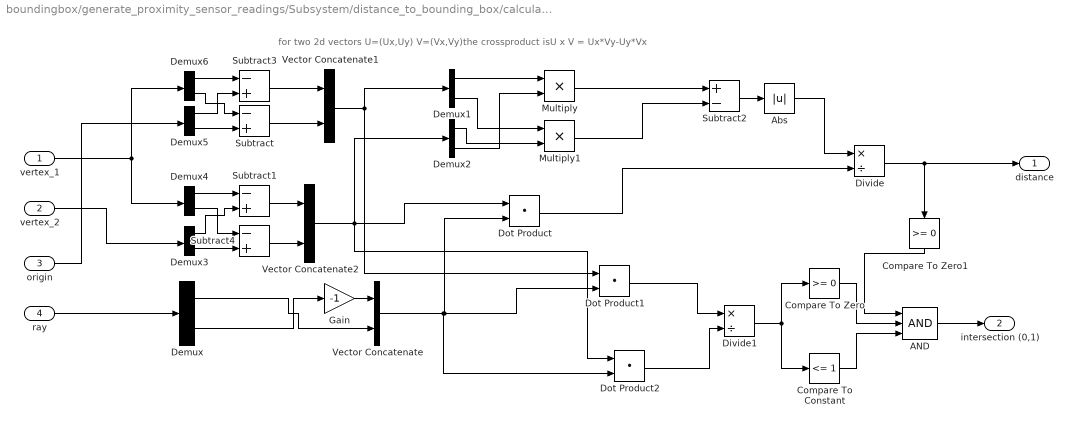
== system boundingbox/generate_proximity_sensor_readings/Subsystem/distance_to_bounding_box/calculate_intersection 2 ==
  note: for two 2d vectors U=(Ux,Uy) V=(Vx,Vy)the crossproduct isU x V = Ux*Vy-Uy*Vx
  vertex_1 : Inport
  vertex_2 : Inport  Port=2
  "origin " : Inport  Port=3
  ray : Inport  Port=4
  AND : Logic  Inputs=3  IconShape=distinctive  AllPortsSameDT=off  OutDataTypeStr=boolean
  Abs : Abs
  Compare To Constant : simulink/Logic and Bit Operations/Compare To Constant  relop=<=  const=1  OutDataTypeStr=boolean
  Compare To Zero : simulink/Logic and Bit Operations/Compare To Zero  relop=>=  OutDataTypeStr=boolean
  Compare To Zero1 : simulink/Logic and Bit Operations/Compare To Zero  relop=>=  OutDataTypeStr=boolean
  Demux{,1..6} (7 alike) : Demux  Outputs=2
  Divide : Product  Inputs=*/
  Divide1 : Product  Inputs=*/
  Dot Product : DotProduct  InputSameDT=on  OutDataTypeStr=Inherit: Inherit via internal rule
  Dot Product1 : DotProduct  InputSameDT=on  OutDataTypeStr=Inherit: Inherit via internal rule
  Dot Product2 : DotProduct  InputSameDT=on  OutDataTypeStr=Inherit: Inherit via internal rule
  Gain : Gain  Gain=-1
  Multiply : Product
  Multiply1 : Product
  Subtract{,1,3..4} (4 alike) : Sum  Inputs=-+
  Subtract2 : Sum  Inputs=+-
  Vector Concatenate : Concatenate
  Vector Concatenate1 : Concatenate
  Vector Concatenate2 : Concatenate
  distance : Outport
  intersection (0,1) : Outport  Port=2
  wires:
  Compare To Constant/1 -> AND/3
  Compare To Zero/1 -> AND/2
  Divide1/1 -> Compare To Zero/1, Compare To Constant/1
  AND/1 -> intersection (0,1)/1
  Dot Product2/1 -> Divide1/2
  Dot Product1/1 -> Divide1/1
  Multiply1/1 -> Subtract2/2
  Multiply/1 -> Subtract2/1
  Demux2/1 -> Multiply1/2
  Demux1/2 -> Multiply1/1
  Demux2/2 -> Multiply/2
  Demux1/1 -> Multiply/1
  Abs/1 -> Divide/1
  Subtract2/1 -> Abs/1
  Dot Product/1 -> Divide/2
  Divide/1 -> Compare To Zero1/1, distance/1
  Subtract/1 -> Vector Concatenate1/2
  Vector Concatenate/1 -> Dot Product/2, Dot Product1/2, Dot Product2/2
  Demux/1 -> Vector Concatenate/2
  Gain/1 -> Vector Concatenate/1
  Demux/2 -> Gain/1
  ray/1 -> Demux/1
  vertex_2/1 -> Demux3/1
  vertex_1/1 -> Demux6/1, Demux4/1
  "origin "/1 -> Demux5/1
  Demux5/1 -> Subtract3/2
  Demux6/1 -> Subtract3/1
  Demux6/2 -> Subtract/1
  Demux5/2 -> Subtract/2
  Demux4/1 -> Subtract1/1
  Demux4/2 -> Subtract4/1
  Demux3/1 -> Subtract1/2
  Demux3/2 -> Subtract4/2
  Subtract3/1 -> Vector Concatenate1/1
  Vector Concatenate1/1 -> Dot Product1/1, Demux1/1
  Subtract4/1 -> Vector Concatenate2/2
  Subtract1/1 -> Vector Concatenate2/1
  Vector Concatenate2/1 -> Dot Product/1, Demux2/1, Dot Product2/1
  Compare To Zero1/1 -> AND/1

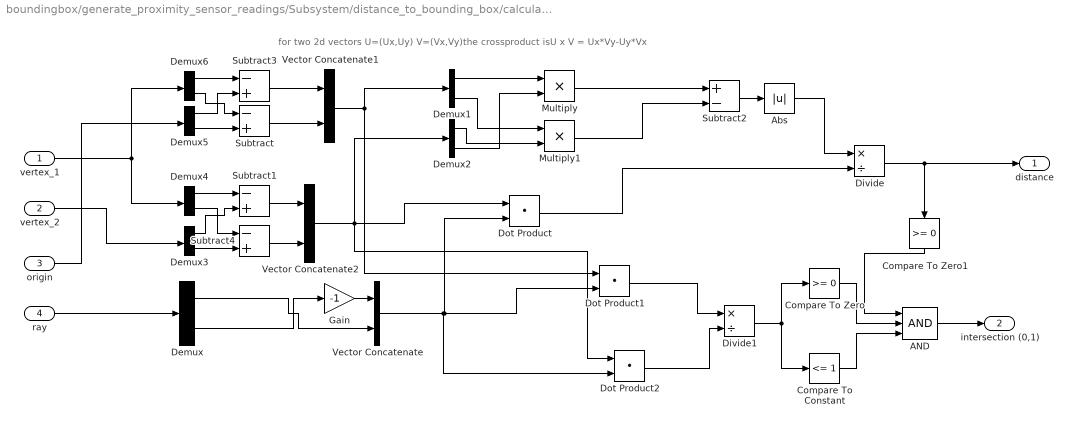
== system boundingbox/generate_proximity_sensor_readings/Subsystem/distance_to_bounding_box/calculate_intersection 3 ==
  note: for two 2d vectors U=(Ux,Uy) V=(Vx,Vy)the crossproduct isU x V = Ux*Vy-Uy*Vx
  vertex_1 : Inport
  vertex_2 : Inport  Port=2
  "origin " : Inport  Port=3
  ray : Inport  Port=4
  AND : Logic  Inputs=3  IconShape=distinctive  AllPortsSameDT=off  OutDataTypeStr=boolean
  Abs : Abs
  Compare To Constant : simulink/Logic and Bit Operations/Compare To Constant  relop=<=  const=1  OutDataTypeStr=boolean
  Compare To Zero : simulink/Logic and Bit Operations/Compare To Zero  relop=>=  OutDataTypeStr=boolean
  Compare To Zero1 : simulink/Logic and Bit Operations/Compare To Zero  relop=>=  OutDataTypeStr=boolean
  Demux{,1..6} (7 alike) : Demux  Outputs=2
  Divide : Product  Inputs=*/
  Divide1 : Product  Inputs=*/
  Dot Product : DotProduct  InputSameDT=on  OutDataTypeStr=Inherit: Inherit via internal rule
  Dot Product1 : DotProduct  InputSameDT=on  OutDataTypeStr=Inherit: Inherit via internal rule
  Dot Product2 : DotProduct  InputSameDT=on  OutDataTypeStr=Inherit: Inherit via internal rule
  Gain : Gain  Gain=-1
  Multiply : Product
  Multiply1 : Product
  Subtract{,1,3..4} (4 alike) : Sum  Inputs=-+
  Subtract2 : Sum  Inputs=+-
  Vector Concatenate : Concatenate
  Vector Concatenate1 : Concatenate
  Vector Concatenate2 : Concatenate
  distance : Outport
  intersection (0,1) : Outport  Port=2
  wires:
  Compare To Zero1/1 -> AND/1
  Vector Concatenate2/1 -> Dot Product2/1, Demux2/1, Dot Product/1
  Subtract1/1 -> Vector Concatenate2/1
  Subtract4/1 -> Vector Concatenate2/2
  Vector Concatenate1/1 -> Demux1/1, Dot Product1/1
  Subtract3/1 -> Vector Concatenate1/1
  Demux3/2 -> Subtract4/2
  Demux3/1 -> Subtract1/2
  Demux4/2 -> Subtract4/1
  Demux4/1 -> Subtract1/1
  Demux5/2 -> Subtract/2
  Demux6/2 -> Subtract/1
  Demux6/1 -> Subtract3/1
  Demux5/1 -> Subtract3/2
  "origin "/1 -> Demux5/1
  vertex_1/1 -> Demux4/1, Demux6/1
  vertex_2/1 -> Demux3/1
  ray/1 -> Demux/1
  Demux/2 -> Gain/1
  Gain/1 -> Vector Concatenate/1
  Demux/1 -> Vector Concatenate/2
  Vector Concatenate/1 -> Dot Product2/2, Dot Product1/2, Dot Product/2
  Subtract/1 -> Vector Concatenate1/2
  Divide/1 -> distance/1, Compare To Zero1/1
  Dot Product/1 -> Divide/2
  Subtract2/1 -> Abs/1
  Abs/1 -> Divide/1
  Demux1/1 -> Multiply/1
  Demux2/2 -> Multiply/2
  Demux1/2 -> Multiply1/1
  Demux2/1 -> Multiply1/2
  Multiply/1 -> Subtract2/1
  Multiply1/1 -> Subtract2/2
  Dot Product1/1 -> Divide1/1
  Dot Product2/1 -> Divide1/2
  AND/1 -> intersection (0,1)/1
  Divide1/1 -> Compare To Constant/1, Compare To Zero/1
  Compare To Zero/1 -> AND/2
  Compare To Constant/1 -> AND/3

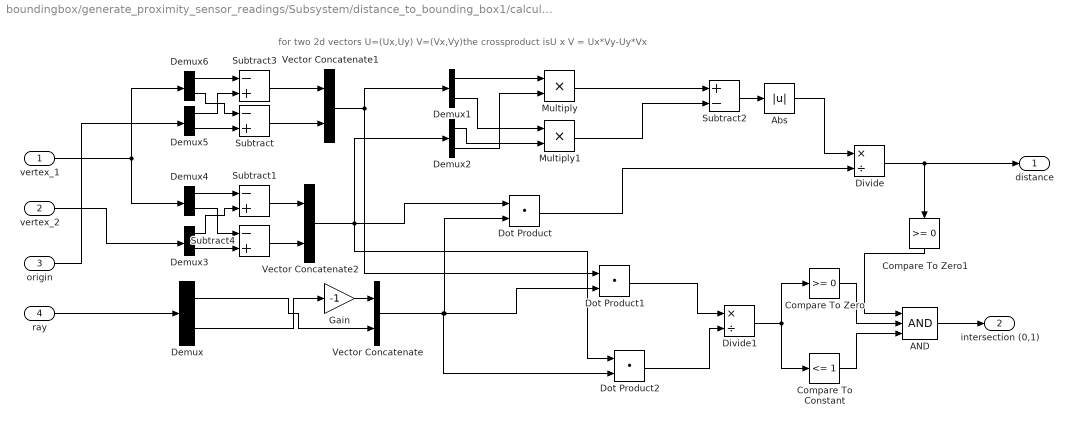
== system boundingbox/generate_proximity_sensor_readings/Subsystem/distance_to_bounding_box1/calculate_intersection  ==
  note: for two 2d vectors U=(Ux,Uy) V=(Vx,Vy)the crossproduct isU x V = Ux*Vy-Uy*Vx
  vertex_1 : Inport
  vertex_2 : Inport  Port=2
  "origin " : Inport  Port=3
  ray : Inport  Port=4
  AND : Logic  Inputs=3  IconShape=distinctive  AllPortsSameDT=off  OutDataTypeStr=boolean
  Abs : Abs
  Compare To Constant : simulink/Logic and Bit Operations/Compare To Constant  relop=<=  const=1  OutDataTypeStr=boolean
  Compare To Zero : simulink/Logic and Bit Operations/Compare To Zero  relop=>=  OutDataTypeStr=boolean
  Compare To Zero1 : simulink/Logic and Bit Operations/Compare To Zero  relop=>=  OutDataTypeStr=boolean
  Demux{,1..6} (7 alike) : Demux  Outputs=2
  Divide : Product  Inputs=*/
  Divide1 : Product  Inputs=*/
  Dot Product : DotProduct  InputSameDT=on  OutDataTypeStr=Inherit: Inherit via internal rule
  Dot Product1 : DotProduct  InputSameDT=on  OutDataTypeStr=Inherit: Inherit via internal rule
  Dot Product2 : DotProduct  InputSameDT=on  OutDataTypeStr=Inherit: Inherit via internal rule
  Gain : Gain  Gain=-1
  Multiply : Product
  Multiply1 : Product
  Subtract{,1,3..4} (4 alike) : Sum  Inputs=-+
  Subtract2 : Sum  Inputs=+-
  Vector Concatenate : Concatenate
  Vector Concatenate1 : Concatenate
  Vector Concatenate2 : Concatenate
  distance : Outport
  intersection (0,1) : Outport  Port=2
  wires:
  Compare To Constant/1 -> AND/3
  Compare To Zero/1 -> AND/2
  Divide1/1 -> Compare To Zero/1, Compare To Constant/1
  AND/1 -> intersection (0,1)/1
  Dot Product2/1 -> Divide1/2
  Dot Product1/1 -> Divide1/1
  Multiply1/1 -> Subtract2/2
  Multiply/1 -> Subtract2/1
  Demux2/1 -> Multiply1/2
  Demux1/2 -> Multiply1/1
  Demux2/2 -> Multiply/2
  Demux1/1 -> Multiply/1
  Abs/1 -> Divide/1
  Subtract2/1 -> Abs/1
  Dot Product/1 -> Divide/2
  Divide/1 -> Compare To Zero1/1, distance/1
  Subtract/1 -> Vector Concatenate1/2
  Vector Concatenate/1 -> Dot Product/2, Dot Product1/2, Dot Product2/2
  Demux/1 -> Vector Concatenate/2
  Gain/1 -> Vector Concatenate/1
  Demux/2 -> Gain/1
  ray/1 -> Demux/1
  vertex_2/1 -> Demux3/1
  vertex_1/1 -> Demux6/1, Demux4/1
  "origin "/1 -> Demux5/1
  Demux5/1 -> Subtract3/2
  Demux6/1 -> Subtract3/1
  Demux6/2 -> Subtract/1
  Demux5/2 -> Subtract/2
  Demux4/1 -> Subtract1/1
  Demux4/2 -> Subtract4/1
  Demux3/1 -> Subtract1/2
  Demux3/2 -> Subtract4/2
  Subtract3/1 -> Vector Concatenate1/1
  Vector Concatenate1/1 -> Dot Product1/1, Demux1/1
  Subtract4/1 -> Vector Concatenate2/2
  Subtract1/1 -> Vector Concatenate2/1
  Vector Concatenate2/1 -> Dot Product/1, Demux2/1, Dot Product2/1
  Compare To Zero1/1 -> AND/1

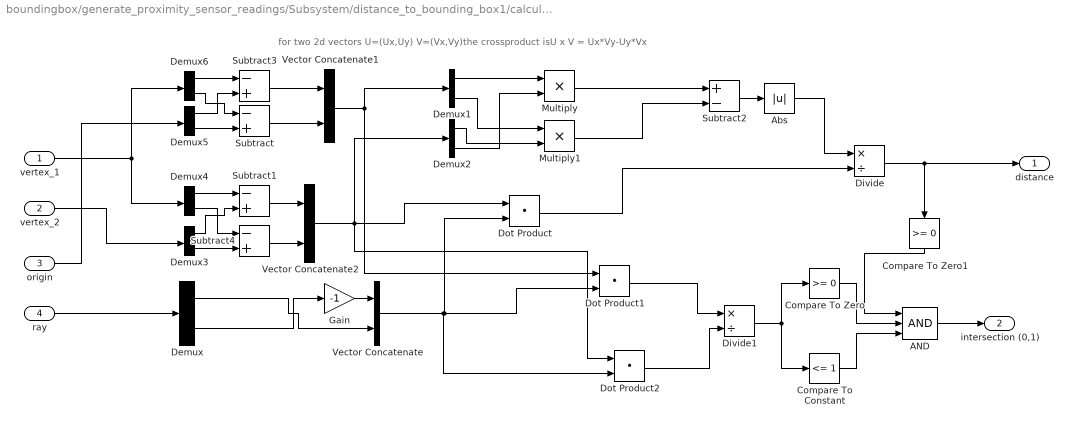
== system boundingbox/generate_proximity_sensor_readings/Subsystem/distance_to_bounding_box1/calculate_intersection 1 ==
  note: for two 2d vectors U=(Ux,Uy) V=(Vx,Vy)the crossproduct isU x V = Ux*Vy-Uy*Vx
  vertex_1 : Inport
  vertex_2 : Inport  Port=2
  "origin " : Inport  Port=3
  ray : Inport  Port=4
  AND : Logic  Inputs=3  IconShape=distinctive  AllPortsSameDT=off  OutDataTypeStr=boolean
  Abs : Abs
  Compare To Constant : simulink/Logic and Bit Operations/Compare To Constant  relop=<=  const=1  OutDataTypeStr=boolean
  Compare To Zero : simulink/Logic and Bit Operations/Compare To Zero  relop=>=  OutDataTypeStr=boolean
  Compare To Zero1 : simulink/Logic and Bit Operations/Compare To Zero  relop=>=  OutDataTypeStr=boolean
  Demux{,1..6} (7 alike) : Demux  Outputs=2
  Divide : Product  Inputs=*/
  Divide1 : Product  Inputs=*/
  Dot Product : DotProduct  InputSameDT=on  OutDataTypeStr=Inherit: Inherit via internal rule
  Dot Product1 : DotProduct  InputSameDT=on  OutDataTypeStr=Inherit: Inherit via internal rule
  Dot Product2 : DotProduct  InputSameDT=on  OutDataTypeStr=Inherit: Inherit via internal rule
  Gain : Gain  Gain=-1
  Multiply : Product
  Multiply1 : Product
  Subtract{,1,3..4} (4 alike) : Sum  Inputs=-+
  Subtract2 : Sum  Inputs=+-
  Vector Concatenate : Concatenate
  Vector Concatenate1 : Concatenate
  Vector Concatenate2 : Concatenate
  distance : Outport
  intersection (0,1) : Outport  Port=2
  wires:
  Compare To Zero1/1 -> AND/1
  Vector Concatenate2/1 -> Dot Product2/1, Demux2/1, Dot Product/1
  Subtract1/1 -> Vector Concatenate2/1
  Subtract4/1 -> Vector Concatenate2/2
  Vector Concatenate1/1 -> Demux1/1, Dot Product1/1
  Subtract3/1 -> Vector Concatenate1/1
  Demux3/2 -> Subtract4/2
  Demux3/1 -> Subtract1/2
  Demux4/2 -> Subtract4/1
  Demux4/1 -> Subtract1/1
  Demux5/2 -> Subtract/2
  Demux6/2 -> Subtract/1
  Demux6/1 -> Subtract3/1
  Demux5/1 -> Subtract3/2
  "origin "/1 -> Demux5/1
  vertex_1/1 -> Demux4/1, Demux6/1
  vertex_2/1 -> Demux3/1
  ray/1 -> Demux/1
  Demux/2 -> Gain/1
  Gain/1 -> Vector Concatenate/1
  Demux/1 -> Vector Concatenate/2
  Vector Concatenate/1 -> Dot Product2/2, Dot Product1/2, Dot Product/2
  Subtract/1 -> Vector Concatenate1/2
  Divide/1 -> distance/1, Compare To Zero1/1
  Dot Product/1 -> Divide/2
  Subtract2/1 -> Abs/1
  Abs/1 -> Divide/1
  Demux1/1 -> Multiply/1
  Demux2/2 -> Multiply/2
  Demux1/2 -> Multiply1/1
  Demux2/1 -> Multiply1/2
  Multiply/1 -> Subtract2/1
  Multiply1/1 -> Subtract2/2
  Dot Product1/1 -> Divide1/1
  Dot Product2/1 -> Divide1/2
  AND/1 -> intersection (0,1)/1
  Divide1/1 -> Compare To Constant/1, Compare To Zero/1
  Compare To Zero/1 -> AND/2
  Compare To Constant/1 -> AND/3

== system boundingbox/generate_proximity_sensor_readings/Subsystem/distance_to_bounding_box1/calculate_intersection 2 ==
  note: for two 2d vectors U=(Ux,Uy) V=(Vx,Vy)the crossproduct isU x V = Ux*Vy-Uy*Vx
  vertex_1 : Inport
  vertex_2 : Inport  Port=2
  "origin " : Inport  Port=3
  ray : Inport  Port=4
  AND : Logic  Inputs=3  IconShape=distinctive  AllPortsSameDT=off  OutDataTypeStr=boolean
  Abs : Abs
  Compare To Constant : simulink/Logic and Bit Operations/Compare To Constant  relop=<=  const=1  OutDataTypeStr=boolean
  Compare To Zero : simulink/Logic and Bit Operations/Compare To Zero  relop=>=  OutDataTypeStr=boolean
  Compare To Zero1 : simulink/Logic and Bit Operations/Compare To Zero  relop=>=  OutDataTypeStr=boolean
  Demux{,1..6} (7 alike) : Demux  Outputs=2
  Divide : Product  Inputs=*/
  Divide1 : Product  Inputs=*/
  Dot Product : DotProduct  InputSameDT=on  OutDataTypeStr=Inherit: Inherit via internal rule
  Dot Product1 : DotProduct  InputSameDT=on  OutDataTypeStr=Inherit: Inherit via internal rule
  Dot Product2 : DotProduct  InputSameDT=on  OutDataTypeStr=Inherit: Inherit via internal rule
  Gain : Gain  Gain=-1
  Multiply : Product
  Multiply1 : Product
  Subtract{,1,3..4} (4 alike) : Sum  Inputs=-+
  Subtract2 : Sum  Inputs=+-
  Vector Concatenate : Concatenate
  Vector Concatenate1 : Concatenate
  Vector Concatenate2 : Concatenate
  distance : Outport
  intersection (0,1) : Outport  Port=2
  wires:
  Compare To Constant/1 -> AND/3
  Compare To Zero/1 -> AND/2
  Divide1/1 -> Compare To Zero/1, Compare To Constant/1
  AND/1 -> intersection (0,1)/1
  Dot Product2/1 -> Divide1/2
  Dot Product1/1 -> Divide1/1
  Multiply1/1 -> Subtract2/2
  Multiply/1 -> Subtract2/1
  Demux2/1 -> Multiply1/2
  Demux1/2 -> Multiply1/1
  Demux2/2 -> Multiply/2
  Demux1/1 -> Multiply/1
  Abs/1 -> Divide/1
  Subtract2/1 -> Abs/1
  Dot Product/1 -> Divide/2
  Divide/1 -> Compare To Zero1/1, distance/1
  Subtract/1 -> Vector Concatenate1/2
  Vector Concatenate/1 -> Dot Product/2, Dot Product1/2, Dot Product2/2
  Demux/1 -> Vector Concatenate/2
  Gain/1 -> Vector Concatenate/1
  Demux/2 -> Gain/1
  ray/1 -> Demux/1
  vertex_2/1 -> Demux3/1
  vertex_1/1 -> Demux6/1, Demux4/1
  "origin "/1 -> Demux5/1
  Demux5/1 -> Subtract3/2
  Demux6/1 -> Subtract3/1
  Demux6/2 -> Subtract/1
  Demux5/2 -> Subtract/2
  Demux4/1 -> Subtract1/1
  Demux4/2 -> Subtract4/1
  Demux3/1 -> Subtract1/2
  Demux3/2 -> Subtract4/2
  Subtract3/1 -> Vector Concatenate1/1
  Vector Concatenate1/1 -> Dot Product1/1, Demux1/1
  Subtract4/1 -> Vector Concatenate2/2
  Subtract1/1 -> Vector Concatenate2/1
  Vector Concatenate2/1 -> Dot Product/1, Demux2/1, Dot Product2/1
  Compare To Zero1/1 -> AND/1

== system boundingbox/generate_proximity_sensor_readings/Subsystem/distance_to_bounding_box1/calculate_intersection 3 ==
  note: for two 2d vectors U=(Ux,Uy) V=(Vx,Vy)the crossproduct isU x V = Ux*Vy-Uy*Vx
  vertex_1 : Inport
  vertex_2 : Inport  Port=2
  "origin " : Inport  Port=3
  ray : Inport  Port=4
  AND : Logic  Inputs=3  IconShape=distinctive  AllPortsSameDT=off  OutDataTypeStr=boolean
  Abs : Abs
  Compare To Constant : simulink/Logic and Bit Operations/Compare To Constant  relop=<=  const=1  OutDataTypeStr=boolean
  Compare To Zero : simulink/Logic and Bit Operations/Compare To Zero  relop=>=  OutDataTypeStr=boolean
  Compare To Zero1 : simulink/Logic and Bit Operations/Compare To Zero  relop=>=  OutDataTypeStr=boolean
  Demux{,1..6} (7 alike) : Demux  Outputs=2
  Divide : Product  Inputs=*/
  Divide1 : Product  Inputs=*/
  Dot Product : DotProduct  InputSameDT=on  OutDataTypeStr=Inherit: Inherit via internal rule
  Dot Product1 : DotProduct  InputSameDT=on  OutDataTypeStr=Inherit: Inherit via internal rule
  Dot Product2 : DotProduct  InputSameDT=on  OutDataTypeStr=Inherit: Inherit via internal rule
  Gain : Gain  Gain=-1
  Multiply : Product
  Multiply1 : Product
  Subtract{,1,3..4} (4 alike) : Sum  Inputs=-+
  Subtract2 : Sum  Inputs=+-
  Vector Concatenate : Concatenate
  Vector Concatenate1 : Concatenate
  Vector Concatenate2 : Concatenate
  distance : Outport
  intersection (0,1) : Outport  Port=2
  wires:
  Compare To Zero1/1 -> AND/1
  Vector Concatenate2/1 -> Dot Product2/1, Demux2/1, Dot Product/1
  Subtract1/1 -> Vector Concatenate2/1
  Subtract4/1 -> Vector Concatenate2/2
  Vector Concatenate1/1 -> Demux1/1, Dot Product1/1
  Subtract3/1 -> Vector Concatenate1/1
  Demux3/2 -> Subtract4/2
  Demux3/1 -> Subtract1/2
  Demux4/2 -> Subtract4/1
  Demux4/1 -> Subtract1/1
  Demux5/2 -> Subtract/2
  Demux6/2 -> Subtract/1
  Demux6/1 -> Subtract3/1
  Demux5/1 -> Subtract3/2
  "origin "/1 -> Demux5/1
  vertex_1/1 -> Demux4/1, Demux6/1
  vertex_2/1 -> Demux3/1
  ray/1 -> Demux/1
  Demux/2 -> Gain/1
  Gain/1 -> Vector Concatenate/1
  Demux/1 -> Vector Concatenate/2
  Vector Concatenate/1 -> Dot Product2/2, Dot Product1/2, Dot Product/2
  Subtract/1 -> Vector Concatenate1/2
  Divide/1 -> distance/1, Compare To Zero1/1
  Dot Product/1 -> Divide/2
  Subtract2/1 -> Abs/1
  Abs/1 -> Divide/1
  Demux1/1 -> Multiply/1
  Demux2/2 -> Multiply/2
  Demux1/2 -> Multiply1/1
  Demux2/1 -> Multiply1/2
  Multiply/1 -> Subtract2/1
  Multiply1/1 -> Subtract2/2
  Dot Product1/1 -> Divide1/1
  Dot Product2/1 -> Divide1/2
  AND/1 -> intersection (0,1)/1
  Divide1/1 -> Compare To Constant/1, Compare To Zero/1
  Compare To Zero/1 -> AND/2
  Compare To Constant/1 -> AND/3
